simulink model "StdAnimation_Runner"  (R2020b)
settings: configuration reference "VLS_SIL_Configuration" (kept outside this file)
settings Model: DataDictionary=StdAnimation_TestingDD.sldd  Creator=mchawa  LastModifiedBy=oashraf
settings ConfigSetRef: SourceName=VLS_SIL_Configuration

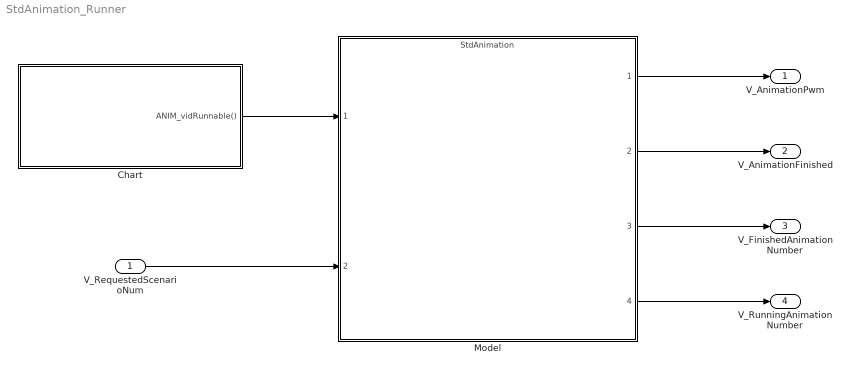
== system StdAnimation_Runner ==
  V_RequestedScenarioNum : Inport
  Chart : Stateflow chart  TreatAsAtomicUnit=on
  Model : ModelReference  ModelNameDialog=StdAnimation.slx  SimulationMode=Normal  ScheduleRates=on  ModelReferenceVersion=1.85
  V_AnimationPwm : Outport
  V_AnimationFinished : Outport  Port=2
  V_FinishedAnimationNumber : Outport  Port=3
  V_RunningAnimationNumber : Outport  Port=4
  wires:
  Chart/1(ANIM_vidRunnable()) -> Model/1
  Model/2 -> V_AnimationFinished/1
  Model/3 -> V_FinishedAnimationNumber/1
  Model/4 -> V_RunningAnimationNumber/1
  V_RequestedScenarioNum/1 -> Model/2
  Model/1 -> V_AnimationPwm/1

== stateflow chart StdAnimation_Runner/Chart ==
  state Scheduler
    on every(1, tick):
    send(ANIM_vidRunnable);
  (default) -> Scheduler
  events: ANIM_vidRunnable output FUNCTION_CALL_EVENT
